simulink model "MySusp_ParasiticStiffness_RTW"  (R2022a)
settings: Solver=ode1  StartTime=0.0  StopTime=inf  FixedStep=0.001  RelTol=1e-3
PreLoadFcn:
  | vehicle = 'Car'; if ~length(which('cmself')), cmenv; end
  | MySusp_ParasiticStiffness_RTW_bus
  | MySusp_ParasiticStiffness_RTW_params
InitFcn:
  | vehicle = 'Car'; if ~length(which('cmself')), cmenv; end
  | MySusp_ParasiticStiffness_RTW_bus
undefined symbols (not defined in the file or in its folder): Coeff
Description:
  | CarMaker Plug-in Model Target
settings Model: Creator=IPG  LastModifiedBy=IPG
settings SolverCC: AlgebraicLoopSolver=TrustRegion
settings DataIOCC: ReturnWorkspaceOutputs=off
settings DebuggingCC: UnconnectedInputMsg=warning  UnconnectedOutputMsg=warning  UnconnectedLineMsg=warning  PregeneratedLibrarySubsystemCodeDiagnostic=none  SFMachineParentedDataDiag=warning  ArithmeticOperatorsInVariantConditions=warning
settings SFSimCC: SimUseLocalCustomCode=off  CustomCodeUndefinedFunction=UseInterfaceOnly
settings RTWCC: Description=CarMaker Plug-in Model Target  SystemTargetFile=CarMaker.tlc  TemplateMakefile=CarMaker_unix-win64.tmf  RTWUseLocalCustomCode=off  DLArmComputeVersion=19.05
settings CodeAppCC: MaxIdLength=127  StateflowObjectComments=on
settings STFCustomTargetCC: TargetLangStandard=C99 (ISO)  CombineOutputUpdateFcns=on  CodeInterfacePackaging=Reusable function  GRTInterface=off  GenerateAllocFcn=on  SystemTargetFile=CarMaker.tlc
settings GRTTargetCC: ParMdlRefBuildCompliant=off  CompOptLevelCompliant=off  ConcurrentExecutionCompliant=off  MatFileLogging=off  CodeInterfacePackaging=Reusable function  CPPClassGenCompliant=off  GenerateAllocFcn=on  UseToolchainInfoCompliant=off  RTWCAPISignals=on  RTWCAPIParams=on  RTWCAPIStates=on

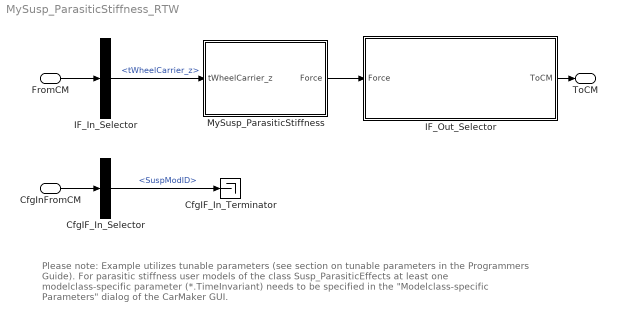
== system MySusp_ParasiticStiffness_RTW ==
  note: Please note: Example utilizes tunable parameters (see section on tunable parameters in the Programmers Guide).
      |
      | For parasitic stiffness user models of the class Susp_ParasiticEffects at least one modelclass-specific parameter (*.TimeInvariant) needs to be specified in the
      | "Modelclass-specific Parameters" dialog of the CarMaker GUI.
  FromCM : Inport  OutDataTypeStr=Bus: cmSusp_ParasiticEffectsIn
  CfgInFromCM : Inport  Port=2  OutDataTypeStr=Bus: cmSusp_ParasiticEffectsCfgIn
  CfgIF_In_Selector : BusSelector  OutputSignals=SuspModID
  CfgIF_In_Terminator : Terminator
  IF_In_Selector : BusSelector  OutputSignals=tWheelCarrier_z
  IF_Out_Selector : Subsystem  mask(Signal Selection){}
      mask help: Signal Selection Block
      settings: OpenFcn=cmSignalSelect('SignalSelection_CB',gcb)
  MySusp_ParasiticStiffness : Subsystem
  ToCM : Outport  OutDataTypeStr=Bus: cmSusp_ParasiticEffectsOut  VectorParamsAs1DForOutWhenUnconnected=off
  wires:
  FromCM/1 -> IF_In_Selector/1
  IF_Out_Selector/1(ToCM) -> ToCM/1
  CfgInFromCM/1 -> CfgIF_In_Selector/1
  CfgIF_In_Selector/1 -> CfgIF_In_Terminator/1  "<SuspModID>"
  IF_In_Selector/1 -> MySusp_ParasiticStiffness/1(tWheelCarrier_z)  "<tWheelCarrier_z>"
  MySusp_ParasiticStiffness/1(Force) -> IF_Out_Selector/1(Force)

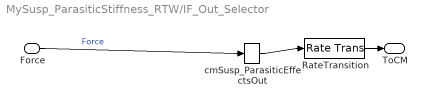
== system MySusp_ParasiticStiffness_RTW/IF_Out_Selector ==
  Force : Inport
  RateTransition : RateTransition  OutPortSampleTime=str2num(get_param(bdroot,'FixedStep'))
  cmSusp_ParasiticEffectsOut : BusCreator  Inputs=1
  ToCM : Outport  VectorParamsAs1DForOutWhenUnconnected=off
  wires:
  RateTransition/1 -> ToCM/1
  cmSusp_ParasiticEffectsOut/1 -> RateTransition/1
  Force/1 -> cmSusp_ParasiticEffectsOut/1  "Force"

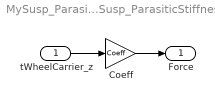
== system MySusp_ParasiticStiffness_RTW/MySusp_ParasiticStiffness ==
  tWheelCarrier_z : Inport
  Coeff : Gain  Gain=Coeff
  Force : Outport  VectorParamsAs1DForOutWhenUnconnected=off
  wires:
  tWheelCarrier_z/1 -> Coeff/1
  Coeff/1 -> Force/1
